simulink library "pwrsys"  (R2018a)
settings: Solver=VariableStepAuto  StartTime=0.0  StopTime=10.0  RelTol=1e-3
values from neighbouring files (symbols this model uses):
  Ts = Ts_c    (= 1e-07)    [PlantStateEquations_abc_Script.m]
undefined symbols (not defined in the file or in its folder): D1, Delta, DiscIntNeverNeededParam, ESS, f_LPF_noise, fn, fsw, grid, gt1, Iap, Kp, PCC, Refmax, Refmin, sim, SIMU, Sn, tctrl, Ti, Ts_control, Ts_PWM, Uabp, Uanp, WT, X, zeta
libraries: $bdroot x71, powerlib x59, powerlib_meascontrol x49, peTransforms x20, PhD_Library x1, sps_avr x1
(part 3 of 4)

== system pwrsys/Transformations/abc_dq ==
  vabc : Inport
  iabc : Inport  Port=2
  wt : Inport  Port=3
  Bus Creator : BusCreator  Inputs=4
  Digital first order LPF : $bdroot/Basic Blocks/Digital first order LPF  Ts=Ts  fcutout=fcutoutv
  Digital first order LPF1 : $bdroot/Basic Blocks/Digital first order LPF  Ts=Ts  fcutout=fcutouti
  Rate Transition1 : RateTransition  OutPortSampleTime=Ts
  Rate Transition2 : RateTransition  OutPortSampleTime=Ts
  Rate Transition4 : RateTransition  OutPortSampleTime=Ts
  Second-Order Filter1 : powerlib_meascontrol/Filters/Second-Order Filter  FilterType=Bandstop (Notch)  Fo=fn  Zeta=zeta  Ts=Ts  Initialize=off  Vac_Init="[0,  0,  60]"  Vdc_Init=0  PlotResponse=off  FreqRange=[0, 1000, 0.1]
      settings: SourceProductName=Simscape Power Systems  SourceProductBaseCode=PS
  Second-Order Filter5 : powerlib_meascontrol/Filters/Second-Order Filter  FilterType=Bandstop (Notch)  Fo=fn  Zeta=zeta  Ts=Ts  Initialize=off  Vac_Init="[0,  0,  60]"  Vdc_Init=0  PlotResponse=off  FreqRange=[0, 1000, 0.1]
      settings: SourceProductName=Simscape Power Systems  SourceProductBaseCode=PS
  Selector4 : Selector  InputPortWidth=3  IndexOptions=Index vector (dialog)  Indices=[1 2]  OutputSizes=1
  Selector5 : Selector  InputPortWidth=3  IndexOptions=Index vector (dialog)  Indices=[1 2]  OutputSizes=1
  abc to dq0 : powerlib_meascontrol/Transformations/abc to dq0  Alignment=90 degrees behind phase A axis
  abc to dq1 : powerlib_meascontrol/Transformations/abc to dq0  Alignment=90 degrees behind phase A axis
  vdq : Outport
  idq : Outport  Port=2
  m : Outport  Port=3
  wires:
  abc to dq1/1 -> Selector4/1
  Selector5/1 -> Digital first order LPF/1, Bus Creator/1  "vdq_unfilt"
  Rate Transition1/1 -> abc to dq0/1
  Rate Transition2/1 -> abc to dq1/2, abc to dq0/2
  Selector4/1 -> Bus Creator/2, Digital first order LPF1/1  "idq_unfilt"
  Rate Transition4/1 -> abc to dq1/1
  abc to dq0/1 -> Selector5/1
  Bus Creator/1 -> m/1
  Second-Order Filter5/1 -> vdq/1, Bus Creator/3  "vdq"
  wt/1 -> Rate Transition2/1
  vabc/1 -> Rate Transition1/1
  iabc/1 -> Rate Transition4/1
  Digital first order LPF1/1 -> Second-Order Filter1/1  "idq"
  Digital first order LPF/1 -> Second-Order Filter5/1  "vdq"
  Second-Order Filter1/1 -> Bus Creator/4, idq/1  "idq"

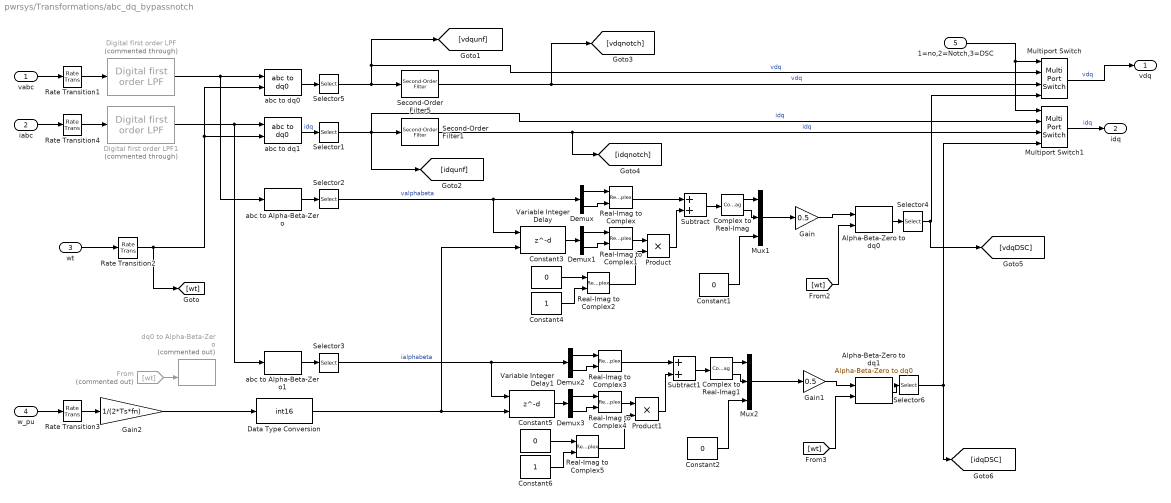
== system pwrsys/Transformations/abc_dq_bypassnotch ==
  vabc : Inport
  iabc : Inport  Port=2
  wt : Inport  Port=3
  w_pu : Inport  Port=4
  1=no,2=Notch,3=DSC : Inport  Port=5
  Alpha-Beta-Zero to dq0 : powerlib_meascontrol/Transformations/Alpha-Beta-Zero to dq0  Alignment=90 degrees behind phase A axis
      settings: SourceProductName=Simscape Power Systems
  Alpha-Beta-Zero to dq1 : powerlib_meascontrol/Transformations/Alpha-Beta-Zero to dq0  Alignment=90 degrees behind phase A axis
      settings: SourceProductName=Simscape Power Systems
  Complex to Real-Imag : ComplexToRealImag
  Complex to Real-Imag1 : ComplexToRealImag
  Constant{1..3,5} (4 alike) : Constant  Value=0
  Constant4 : Constant
  Constant6 : Constant
  Data Type Conversion : DataTypeConversion  OutDataTypeStr=int16  RndMeth=Round  SaturateOnIntegerOverflow=on
  Demux{,1..3} (4 alike) : Demux  Outputs=2
  Digital first order LPF : $bdroot/Basic Blocks/Digital first order LPF  Commented=through  Ts=Ts  fcutout=fcutoutv
  Digital first order LPF1 : $bdroot/Basic Blocks/Digital first order LPF  Commented=through  Ts=Ts  fcutout=fcutouti
  From : From  Commented=on  GotoTag=wt
  Gain : Gain  Gain=0.5
  Gain1 : Gain  Gain=0.5
  Gain2 : Gain  Gain=1/(2*Ts*fn)
  Multiport Switch : MultiPortSwitch
  Multiport Switch1 : MultiPortSwitch
  Mux1 : Mux  Inputs=[1 1 1]
  Mux2 : Mux  Inputs=[1 1 1]
  Product : Product
  Product1 : Product
  Rate Transition1 : RateTransition  OutPortSampleTime=Ts
  Rate Transition2 : RateTransition  OutPortSampleTime=Ts
  Rate Transition3 : RateTransition  InitialCondition=1  OutPortSampleTime=Ts
  Rate Transition4 : RateTransition  OutPortSampleTime=Ts
  Real-Imag to Complex{,1..5} (6 alike) : RealImagToComplex
  Second-Order Filter1 : powerlib_meascontrol/Filters/Second-Order Filter  FilterType=Bandstop (Notch)  Fo=fn  Zeta=zeta  Ts=Ts  Initialize=off  Vac_Init="[0,  0,  60]"  Vdc_Init=0  PlotResponse=off  FreqRange=[0, 1000, 0.1]
      settings: SourceProductName=Simscape Power Systems  SourceProductBaseCode=PS
  Second-Order Filter5 : powerlib_meascontrol/Filters/Second-Order Filter  FilterType=Bandstop (Notch)  Fo=fn  Zeta=zeta  Ts=Ts  Initialize=off  Vac_Init="[0,  0,  60]"  Vdc_Init=0  PlotResponse=off  FreqRange=[0, 1000, 0.1]
      settings: SourceProductName=Simscape Power Systems  SourceProductBaseCode=PS
  Selector{1..6} (6 alike) : Selector  InputPortWidth=3  IndexOptions=Index vector (dialog)  Indices=[1 2]  OutputSizes=1
  Subtract : Sum
  Subtract1 : Sum
  Variable Integer Delay : Delay  DelayLengthSource=Input port  DelayLength=200  DelayLengthUpperLimit=500  SampleTime=Ts
      settings: InputPortMap=u0,p1
  Variable Integer Delay1 : Delay  DelayLengthSource=Input port  DelayLength=200  DelayLengthUpperLimit=500  SampleTime=Ts
      settings: InputPortMap=u0,p1
  abc to Alpha-Beta-Zero : powerlib_meascontrol/Transformations/abc to Alpha-Beta-Zero
      settings: SourceProductName=Simscape Power Systems
  abc to Alpha-Beta-Zero1 : powerlib_meascontrol/Transformations/abc to Alpha-Beta-Zero
      settings: SourceProductName=Simscape Power Systems
  abc to dq0 : powerlib_meascontrol/Transformations/abc to dq0  Alignment=90 degrees behind phase A axis
  abc to dq1 : powerlib_meascontrol/Transformations/abc to dq0  Alignment=90 degrees behind phase A axis
  dq0 to Alpha-Beta-Zero : powerlib_meascontrol/Transformations/dq0 to Alpha-Beta-Zero  Commented=on  Alignment=90 degrees behind phase A axis
      settings: SourceProductName=Simscape Power Systems  SourceProductBaseCode=PS
  vdq : Outport
  idq : Outport  Port=2
  wires:
  Rate Transition1/1 -> Digital first order LPF/1
  Rate Transition2/1 -> [wt], abc to dq1/2, abc to dq0/2
  Rate Transition4/1 -> Digital first order LPF1/1
  wt/1 -> Rate Transition2/1
  abc to dq1/1 -> Selector1/1  "idq"
  Selector5/1 -> Second-Order Filter5/1, [vdqunf], Multiport Switch/2  "vdq"
  Second-Order Filter5/1 -> [vdqnotch], Multiport Switch/3  "vdq"
  Second-Order Filter1/1 -> [idqnotch], Multiport Switch1/3  "idq"
  abc to dq0/1 -> Selector5/1
  Selector1/1 -> [idqunf], Second-Order Filter1/1, Multiport Switch1/2  "idq"
  abc to Alpha-Beta-Zero/1 -> Selector2/1
  abc to Alpha-Beta-Zero1/1 -> Selector3/1
  Gain2/1 -> Data Type Conversion/1
  From/1 -> dq0 to Alpha-Beta-Zero/2
  [wt] -> Alpha-Beta-Zero to dq0/2
  Alpha-Beta-Zero to dq0/1 -> Selector4/1
  Selector4/1 -> [vdqDSC], Multiport Switch/4
  Selector6/1 -> [idqDSC], Multiport Switch1/4
  [wt] -> Alpha-Beta-Zero to dq1/2
  Selector3/1 -> Demux2/1, Variable Integer Delay1/1  "ialphabeta"
  Alpha-Beta-Zero to dq1/1 -> Selector6/1
  Gain/1 -> Alpha-Beta-Zero to dq0/1
  Gain1/1 -> Alpha-Beta-Zero to dq1/1
  Variable Integer Delay/1 -> Demux1/1
  Constant1/1 -> Mux1/3
  Complex to Real-Imag/2 -> Mux1/2
  Constant4/1 -> Real-Imag to Complex2/2
  Complex to Real-Imag/1 -> Mux1/1
  Subtract/1 -> Complex to Real-Imag/1
  Real-Imag to Complex/1 -> Subtract/1
  Demux1/2 -> Real-Imag to Complex1/2
  Real-Imag to Complex1/1 -> Product/1
  Product/1 -> Subtract/2
  Real-Imag to Complex2/1 -> Product/2
  Constant3/1 -> Real-Imag to Complex2/1
  Demux1/1 -> Real-Imag to Complex1/1
  Demux/2 -> Real-Imag to Complex/2
  Demux/1 -> Real-Imag to Complex/1
  Selector2/1 -> Demux/1, Variable Integer Delay/1  "valphabeta"
  Mux1/1 -> Gain/1
  Mux2/1 -> Gain1/1
  Demux2/1 -> Real-Imag to Complex3/1
  Constant5/1 -> Real-Imag to Complex5/1
  Real-Imag to Complex5/1 -> Product1/2
  Demux3/1 -> Real-Imag to Complex4/1
  Product1/1 -> Subtract1/2
  Demux2/2 -> Real-Imag to Complex3/2
  Demux3/2 -> Real-Imag to Complex4/2
  Real-Imag to Complex3/1 -> Subtract1/1
  Constant6/1 -> Real-Imag to Complex5/2
  Real-Imag to Complex4/1 -> Product1/1
  Complex to Real-Imag1/1 -> Mux2/1
  Constant2/1 -> Mux2/3
  Complex to Real-Imag1/2 -> Mux2/2
  Variable Integer Delay1/1 -> Demux3/1
  Subtract1/1 -> Complex to Real-Imag1/1
  Digital first order LPF/1 -> abc to Alpha-Beta-Zero/1, abc to dq0/1
  Digital first order LPF1/1 -> abc to Alpha-Beta-Zero1/1, abc to dq1/1
  w_pu/1 -> Rate Transition3/1
  Rate Transition3/1 -> Gain2/1
  vabc/1 -> Rate Transition1/1
  iabc/1 -> Rate Transition4/1
  Data Type Conversion/1 -> Variable Integer Delay1/2, Variable Integer Delay/2
  Multiport Switch/1 -> vdq/1  "vdq"
  Multiport Switch1/1 -> idq/1  "idq"
  1=no,2=Notch,3=DSC/1 -> Multiport Switch1/1, Multiport Switch/1

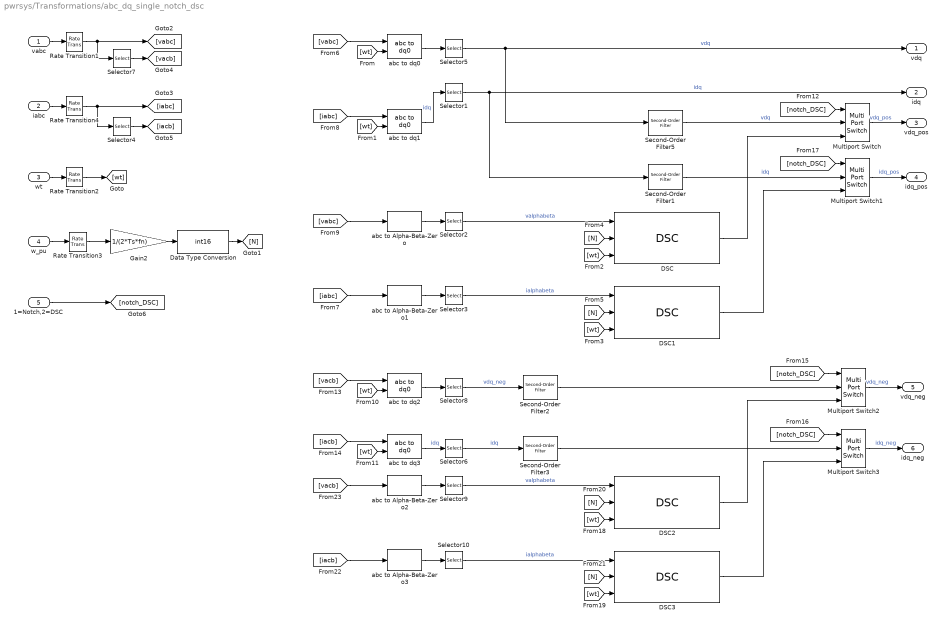
== system pwrsys/Transformations/abc_dq_single_notch_dsc ==
  vabc : Inport
  iabc : Inport  Port=2
  wt : Inport  Port=3
  w_pu : Inport  Port=4
  1=Notch,2=DSC : Inport  Port=5
  DSC{,1..3} (4 alike) : $bdroot/Basic Blocks/DSC
  Data Type Conversion : DataTypeConversion  OutDataTypeStr=int16  RndMeth=Round  SaturateOnIntegerOverflow=on
  Gain2 : Gain  Gain=1/(2*Ts*fn)
  Multiport Switch{,1..3} (4 alike) : MultiPortSwitch  Inputs=2
  Rate Transition1 : RateTransition  OutPortSampleTime=Ts
  Rate Transition2 : RateTransition  OutPortSampleTime=Ts
  Rate Transition3 : RateTransition  InitialCondition=1  OutPortSampleTime=Ts
  Rate Transition4 : RateTransition  OutPortSampleTime=Ts
  Second-Order Filter{1..3,5} (4 alike) : powerlib_meascontrol/Filters/Second-Order Filter  FilterType=Bandstop (Notch)  Fo=fn  Zeta=zeta  Ts=Ts  Initialize=off  Vac_Init="[0,  0,  60]"  Vdc_Init=0  PlotResponse=off  FreqRange=[0, 1000, 0.1]
      settings: SourceProductName=Simscape Power Systems  SourceProductBaseCode=PS
  Selector{1..3,5..6,8..10} (8 alike) : Selector  InputPortWidth=3  IndexOptions=Index vector (dialog)  Indices=[1 2]  OutputSizes=1
  Selector4 : Selector  InputPortWidth=3  IndexOptions=Index vector (dialog)  Indices=[1 3 2]  OutputSizes=1
  Selector7 : Selector  InputPortWidth=3  IndexOptions=Index vector (dialog)  Indices=[1 3 2]  OutputSizes=1
  abc to Alpha-Beta-Zero{,1..3} (4 alike) : powerlib_meascontrol/Transformations/abc to Alpha-Beta-Zero
      settings: SourceProductName=Simscape Power Systems
  abc to dq{0..3} (4 alike) : powerlib_meascontrol/Transformations/abc to dq0  Alignment=90 degrees behind phase A axis
  vdq : Outport
  idq : Outport  Port=2
  vdq_pos : Outport  Port=3
  idq_pos : Outport  Port=4
  vdq_neg : Outport  Port=5
  idq_neg : Outport  Port=6
  wires:
  wt/1 -> Rate Transition2/1
  abc to dq1/1 -> Selector1/1  "idq"
  Selector5/1 -> vdq/1, Second-Order Filter5/1  "vdq"
  abc to dq0/1 -> Selector5/1
  Selector1/1 -> idq/1, Second-Order Filter1/1  "idq"
  abc to Alpha-Beta-Zero/1 -> Selector2/1
  abc to Alpha-Beta-Zero1/1 -> Selector3/1
  Gain2/1 -> Data Type Conversion/1
  DSC/1 -> Multiport Switch/3
  Selector3/1 -> DSC1/1  "ialphabeta"
  [vabc] -> abc to dq0/1
  [iabc] -> abc to dq1/1
  w_pu/1 -> Rate Transition3/1
  Rate Transition3/1 -> Gain2/1
  vabc/1 -> Rate Transition1/1
  iabc/1 -> Rate Transition4/1
  Selector2/1 -> DSC/1  "valphabeta"
  Second-Order Filter5/1 -> Multiport Switch/2  "vdq"
  Second-Order Filter1/1 -> Multiport Switch1/2  "idq"
  DSC1/1 -> Multiport Switch1/3
  Multiport Switch/1 -> vdq_pos/1  "vdq_pos"
  Multiport Switch1/1 -> idq_pos/1  "idq_pos"
  Rate Transition2/1 -> [wt]
  [wt] -> abc to dq0/2
  [wt] -> abc to dq1/2
  [wt] -> DSC/3
  [wt] -> DSC1/3
  [N] -> DSC/2
  [N] -> DSC1/2
  Data Type Conversion/1 -> [N]
  Rate Transition1/1 -> Selector7/1, [vabc]
  Selector7/1 -> [vacb]
  Rate Transition4/1 -> Selector4/1, [iabc]
  Selector4/1 -> [iacb]
  [vabc] -> abc to Alpha-Beta-Zero/1
  [iabc] -> abc to Alpha-Beta-Zero1/1
  [wt] -> abc to dq3/2
  abc to dq2/1 -> Selector8/1
  Selector8/1 -> Second-Order Filter2/1  "vdq_neg"
  [vacb] -> abc to dq2/1
  [wt] -> abc to dq2/2
  abc to dq3/1 -> Selector6/1  "idq"
  [iacb] -> abc to dq3/1
  1=Notch,2=DSC/1 -> [notch_DSC]
  Multiport Switch2/1 -> vdq_neg/1  "vdq_neg"
  Multiport Switch3/1 -> idq_neg/1  "idq_neg"
  Second-Order Filter2/1 -> Multiport Switch2/2
  [notch_DSC] -> Multiport Switch2/1
  [notch_DSC] -> Multiport Switch3/1
  [notch_DSC] -> Multiport Switch/1
  [notch_DSC] -> Multiport Switch1/1
  Selector6/1 -> Second-Order Filter3/1  "idq"
  Second-Order Filter3/1 -> Multiport Switch3/2
  abc to Alpha-Beta-Zero3/1 -> Selector10/1
  Selector10/1 -> DSC3/1  "ialphabeta"
  abc to Alpha-Beta-Zero2/1 -> Selector9/1
  [iacb] -> abc to Alpha-Beta-Zero3/1
  [wt] -> DSC2/3
  [vacb] -> abc to Alpha-Beta-Zero2/1
  DSC2/1 -> Multiport Switch2/3
  Selector9/1 -> DSC2/1  "valphabeta"
  [N] -> DSC3/2
  [N] -> DSC2/2
  DSC3/1 -> Multiport Switch3/3
  [wt] -> DSC3/3

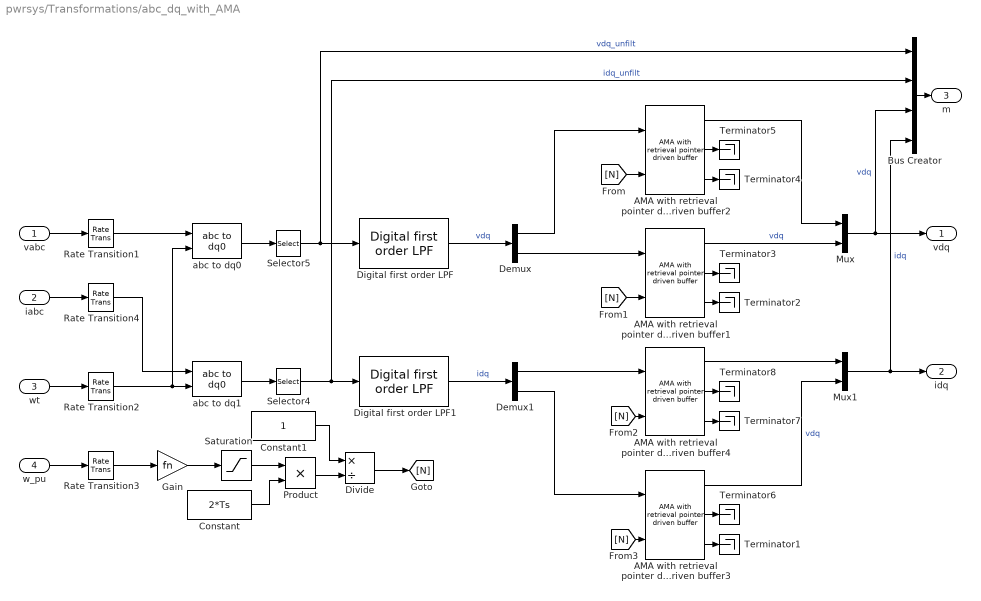
== system pwrsys/Transformations/abc_dq_with_AMA ==
  vabc : Inport
  iabc : Inport  Port=2
  wt : Inport  Port=3
  w_pu : Inport  Port=4
  AMA with retrieval pointer driven buffer{1..4} (4 alike) : $bdroot/Adaptive Moving Averages/AMA with retrieval pointer driven buffer  NbSize=1/(2*fmin*Ts)  Ts=Ts
  Bus Creator : BusCreator  Inputs=4
  Constant : Constant  Value=2*Ts
  Constant1 : Constant
  Demux : Demux  Outputs=2
  Demux1 : Demux  Outputs=2
  Digital first order LPF : $bdroot/Basic Blocks/Digital first order LPF  Ts=Ts  fcutout=fcutoutv
  Digital first order LPF1 : $bdroot/Basic Blocks/Digital first order LPF  Ts=Ts  fcutout=fcutouti
  Divide : Product  Inputs=*/
  Gain : Gain  Gain=fn
  Mux : Mux  Inputs=2
  Mux1 : Mux  Inputs=2
  Product : Product
  Rate Transition1 : RateTransition  OutPortSampleTime=Ts
  Rate Transition2 : RateTransition  OutPortSampleTime=Ts
  Rate Transition3 : RateTransition  InitialCondition=1  OutPortSampleTime=Ts
  Rate Transition4 : RateTransition  OutPortSampleTime=Ts
  Saturation : Saturate  UpperLimit=fmax  LowerLimit=fmin
  Selector4 : Selector  InputPortWidth=3  IndexOptions=Index vector (dialog)  Indices=[1 2]  OutputSizes=1
  Selector5 : Selector  InputPortWidth=3  IndexOptions=Index vector (dialog)  Indices=[1 2]  OutputSizes=1
  Terminator{1..8} (8 alike) : Terminator
  abc to dq0 : powerlib_meascontrol/Transformations/abc to dq0  Alignment=90 degrees behind phase A axis
  abc to dq1 : powerlib_meascontrol/Transformations/abc to dq0  Alignment=90 degrees behind phase A axis
  vdq : Outport
  idq : Outport  Port=2
  m : Outport  Port=3
  wires:
  Digital first order LPF/1 -> Demux/1  "vdq"
  abc to dq1/1 -> Selector4/1
  Mux1/1 -> Bus Creator/4, idq/1  "idq"
  Selector5/1 -> Digital first order LPF/1, Bus Creator/1  "vdq_unfilt"
  Rate Transition1/1 -> abc to dq0/1
  Rate Transition2/1 -> abc to dq0/2, abc to dq1/2
  Selector4/1 -> Bus Creator/2, Digital first order LPF1/1  "idq_unfilt"
  Rate Transition4/1 -> abc to dq1/1
  abc to dq0/1 -> Selector5/1
  Bus Creator/1 -> m/1
  Mux/1 -> Bus Creator/3, vdq/1  "vdq"
  wt/1 -> Rate Transition2/1
  vabc/1 -> Rate Transition1/1
  iabc/1 -> Rate Transition4/1
  AMA with retrieval pointer driven buffer1/3 -> Terminator2/1
  AMA with retrieval pointer driven buffer1/2 -> Terminator3/1
  w_pu/1 -> Rate Transition3/1
  Rate Transition3/1 -> Gain/1
  Gain/1 -> Saturation/1
  Saturation/1 -> Product/1
  Constant/1 -> Product/2
  Product/1 -> Divide/2
  Constant1/1 -> Divide/1
  Divide/1 -> [N]
  Demux/1 -> AMA with retrieval pointer driven buffer2/1
  Demux/2 -> AMA with retrieval pointer driven buffer1/1
  AMA with retrieval pointer driven buffer2/3 -> Terminator4/1
  AMA with retrieval pointer driven buffer2/2 -> Terminator5/1
  AMA with retrieval pointer driven buffer2/1 -> Mux/1
  AMA with retrieval pointer driven buffer1/1 -> Mux/2  "vdq"
  AMA with retrieval pointer driven buffer3/1 -> Mux1/2  "vdq"
  AMA with retrieval pointer driven buffer4/2 -> Terminator8/1
  Demux1/1 -> AMA with retrieval pointer driven buffer4/1
  Demux1/2 -> AMA with retrieval pointer driven buffer3/1
  AMA with retrieval pointer driven buffer4/3 -> Terminator7/1
  AMA with retrieval pointer driven buffer3/3 -> Terminator1/1
  AMA with retrieval pointer driven buffer4/1 -> Mux1/1
  AMA with retrieval pointer driven buffer3/2 -> Terminator6/1
  Digital first order LPF1/1 -> Demux1/1  "idq"
  [N] -> AMA with retrieval pointer driven buffer2/2
  [N] -> AMA with retrieval pointer driven buffer1/2
  [N] -> AMA with retrieval pointer driven buffer4/2
  [N] -> AMA with retrieval pointer driven buffer3/2

== system pwrsys/Transformations/dqz to xyz ==
  note: Inverse Park transform
  dqz : Inport
  scwt : Inport  Port=2
  Demux : Demux  Outputs=3
  Demux1 : Demux  Outputs=2
  Mux : Mux  Inputs=3
  Product{4..7} (4 alike) : Product
  Sum1 : Sum  Inputs=+-
  Sum2 : Sum
  xyz : Outport
  wires:
  dqz/1 -> Demux/1
  Demux/1 -> Product7/2, Product4/2  "d"
  Demux1/2 -> Product4/1, Product6/1
  Product5/1 -> Sum1/2
  Product4/1 -> Sum1/1
  Demux1/1 -> Product7/1, Product5/2
  Demux/2 -> Product6/2, Product5/1  "q"
  scwt/1 -> Demux1/1
  Product6/1 -> Sum2/1
  Product7/1 -> Sum2/2
  Mux/1 -> xyz/1
  Demux/3 -> Mux/3  "z"
  Sum2/1 -> Mux/2  "y"
  Sum1/1 -> Mux/1  "x"

== system pwrsys/Transformations/xyz to abc ==
  note: Inverse Clark Transform
  xyz : Inport
  Demux : Demux  Outputs=3
  Gain : Gain  Gain=d
  Gain1 : Gain  Gain=c
  Gain2 : Gain  Gain=b
  Gain3 : Gain  Gain=a
  Mux : Mux  Inputs=3
  Sum3 : Sum  Inputs=-+
  Sum4 : Sum  Inputs=-+
  Sum5 : Sum
  Sum6 : Sum
  abc : Outport
  wires:
  xyz/1 -> Demux/1
  Demux/2 -> Gain2/1  "y"
  Demux/1 -> Gain3/1, Gain1/1  "x"
  Demux/3 -> Gain/1  "z"
  Gain1/1 -> Sum3/1
  Gain/1 -> Sum6/2, Sum3/2  "A"
  Gain2/1 -> Sum5/1, Sum4/1
  Sum3/1 -> Sum5/2, Sum4/2  "B"
  Sum4/1 -> Mux/3  "c"
  Sum5/1 -> Mux/2  "b"
  Sum6/1 -> Mux/1  "a"
  Gain3/1 -> Sum6/1
  Mux/1 -> abc/1

== system pwrsys/Transformations/xyz to dqz ==
  note: Park transform
  xyz : Inport
  scwt : Inport  Port=2
  Demux : Demux  Outputs=3
  Demux1 : Demux  Outputs=2
  Mux : Mux  Inputs=3
  Product{4..7} (4 alike) : Product
  Sum1 : Sum
  Sum2 : Sum  Inputs=+-
  dqz : Outport
  wires:
  Sum1/1 -> Mux/1  "d"
  Sum2/1 -> Mux/2  "q"
  Demux/3 -> Mux/3  "z"
  Mux/1 -> dqz/1
  Product7/1 -> Sum2/2
  Product6/1 -> Sum2/1
  scwt/1 -> Demux1/1
  Demux/2 -> Product5/1, Product6/2  "y"
  Demux1/1 -> Product5/2, Product7/1
  Product4/1 -> Sum1/1
  Product5/1 -> Sum1/2
  Demux1/2 -> Product6/1, Product4/1
  Demux/1 -> Product4/2, Product7/2  "x"
  xyz/1 -> Demux/1

== system pwrsys/Voltage Sources/Balanced_3_phase_Vsource ==
  amp_pu : Inport
  time_s : Inport  Port=2
  phase_deg : Inport  Port=3
  pos1_neg-1 : Inport  Port=4
  f_pu : Inport  Port=5
  Add3 : Sum  Inputs=+-+
  Add4 : Sum  Inputs=+++
  Add5 : Sum
  Amplitude_Base : Constant  Value=BaseAmp
  Bus Creator : BusCreator  Inputs=3
  Constant : Constant  Value=2*pi
  Constant4 : Constant  Value=2*pi/3
  Constant6 : Constant  Value=2*pi
  Controlled Voltage Source : powerlib/Electrical Sources/Controlled Voltage Source  Initialize=off  Source_Type=AC  Amplitude=ESS.LSC.Ub*(2/3)^0.5  Phase=0  Frequency=PCC.fn  Measurements=None
  Controlled Voltage Source1 : powerlib/Electrical Sources/Controlled Voltage Source  Initialize=off  Source_Type=AC  Amplitude=ESS.LSC.Ub*(2/3)^0.5  Phase=-120  Frequency=PCC.fn  Measurements=None
  Controlled Voltage Source2 : powerlib/Electrical Sources/Controlled Voltage Source  Initialize=off  Source_Type=AC  Amplitude=ESS.LSC.Ub*(2/3)^0.5  Phase=120  Frequency=PCC.fn  Measurements=None
  Gain : Gain  Gain=pi/180
  Gain1 : Gain  Gain=fn
  Product{1,3..5,8} (5 alike) : Product
  Product2 : Product  Inputs=3
  Relay : Relay  OnSwitchValue=0  OffSwitchValue=-0.1  OffOutputValue=-1
  Trigonometric Function3 : Trigonometry
  Trigonometric Function4 : Trigonometry
  Trigonometric Function5 : Trigonometry
  mod : Math  Operator=mod  SaturateOnIntegerOverflow=on
  Va+ : PMIOPort  Side=Right
  Vb+ : PMIOPort  Port=2  Side=Right
  Vc+ : PMIOPort  Port=3  Side=Right
  Va- : PMIOPort  Port=4  Side=Right
  Vb- : PMIOPort  Port=5  Side=Right
  Vc- : PMIOPort  Port=6  Side=Right
  Amp_V : Outport
  phase_rad : Outport  Port=2
  wt_phase_a : Outport  Port=3
  Vabc : Outport  Port=4
  wires:
  Add4/1 -> Trigonometric Function5/1
  Gain/1 -> phase_rad/1, Add4/3, Add3/3, Add5/2  "phase"
  Add3/1 -> Trigonometric Function4/1
  pos1_neg-1/1 -> Relay/1
  Product3/1 -> Bus Creator/1, Controlled Voltage Source/1  "Va"
  amp_pu/1 -> Product1/1
  Product8/1 -> Add3/2, Add4/2
  Product5/1 -> Bus Creator/3, Controlled Voltage Source2/1  "Vc"
  Product4/1 -> Bus Creator/2, Controlled Voltage Source1/1  "Vb"
  Amplitude_Base/1 -> Product1/2
  Constant4/1 -> Product8/1
  Product1/1 -> Product5/1, Product4/1, Product3/1, Amp_V/1  "amp"
  Relay/1 -> Product8/2
  Trigonometric Function3/1 -> Product3/2
  Product2/1 -> Add5/1, Add4/1, Add3/1  "wt"
  Trigonometric Function5/1 -> Product5/2
  Add5/1 -> mod/1, Trigonometric Function3/1
  Trigonometric Function4/1 -> Product4/2
  phase_deg/1 -> Gain/1
  time_s/1 -> Product2/2
  Constant/1 -> Product2/1
  f_pu/1 -> Gain1/1
  Gain1/1 -> Product2/3
  Bus Creator/1 -> Vabc/1
  Constant6/1 -> mod/2
  mod/1 -> wt_phase_a/1
  connections:
  Vb+/RConn1 -- Controlled Voltage Source1/RConn1
  Vc+/RConn1 -- Controlled Voltage Source2/RConn1
  Va+/RConn1 -- Controlled Voltage Source/RConn1
  Va-/RConn1 -- Controlled Voltage Source/LConn1
  Vb-/RConn1 -- Controlled Voltage Source1/LConn1
  Vc-/RConn1 -- Controlled Voltage Source2/LConn1

== system pwrsys/Voltage Sources/DCL_LSC_LCL_Trafo_NoSwitching ==
  Open_Close_Breaker : Inport
  Vabcref : Inport  Port=2
  Bus Creator : BusCreator  Inputs=8
  Cdclink : powerlib/Elements/Parallel RLC Branch  LConnTagsString=a  RConnTagsString=__new0  BranchType=RC  Resistance=1e6  Inductance=0  SetiL0=off  InitialCurrent=0  Capacitance=Cdc  Setx0=on  InitialVoltage=Udc0  Measurements=None
  Controlled Current Source2 : powerlib/Electrical Sources/Controlled Current Source  Initialize=on  Source_Type=DC  Amplitude=0  Phase=0  Frequency=50  Measurements=None
  Controlled Voltage Source : powerlib/Electrical Sources/Controlled Voltage Source  Initialize=on  Source_Type=AC  Amplitude=Uab*(2/3)^0.5  Phase=30  Frequency=fn  Measurements=None
  Controlled Voltage Source1 : powerlib/Electrical Sources/Controlled Voltage Source  Initialize=on  Source_Type=AC  Amplitude=Uab*(2/3)^0.5  Phase=30-120  Frequency=fn  Measurements=None
  Controlled Voltage Source2 : powerlib/Electrical Sources/Controlled Voltage Source  Initialize=on  Source_Type=AC  Amplitude=Uab*(2/3)^0.5  Phase=30+120  Frequency=fn  Measurements=None
  Current Measurement : powerlib/Measurements/Current Measurement  PhasorSimulation=off  OutputType=Complex  PSBequivalent=0
  Demux2 : Demux  Outputs=3
  Divide : Product  Inputs=**/
  Dot Product : DotProduct  InputSameDT=on  OutDataTypeStr=Inherit: Inherit via internal rule
  HV : powerlib/Measurements/Three-Phase V-I Measurement  VoltageMeasurement=phase-to-ground  SetLabelV=off  LabelV=vgrid  Vpu=off  VpuLL=off  CurrentMeasurement=yes  SetLabelI=off  LabelI=igrid  Ipu=off  Pbase=sn  Vbase=uab  OutputType=Complex  PhasorSimulation=off  PSBequivalent=0
  High Res Grounding : powerlib/Elements/Three-Phase Parallel RLC Load  LConnTagsString=A|B|C  Configuration=Y (grounded)  NominalVoltage=Uab  Vabc=[1e3 1e3 1e3]  Vabcp=[1e3 1e3 1e3]  NominalFrequency=fn  UnbalancedPower=off  ActivePower=0.001  InductivePower=0  CapacitivePower=0  Pabc=[10e3 9e3 11e3]  QLabc=[100 90 110]  QCabc=[100 90 110]  Pabcp=[10e3 9e3 11e3]  QLabcp=[100 90 110]  QCabcp=[100 90 110]  Measurements=None  LoadType=constant Z
  INV : powerlib/Measurements/Three-Phase V-I Measurement  VoltageMeasurement=phase-to-ground  SetLabelV=off  LabelV=vconv  Vpu=off  VpuLL=off  CurrentMeasurement=yes  SetLabelI=off  LabelI=iconv  Ipu=off  Pbase=sn  Vbase=uab  OutputType=Complex  PhasorSimulation=off  PSBequivalent=0
  LV : powerlib/Measurements/Three-Phase V-I Measurement  VoltageMeasurement=phase-to-ground  SetLabelV=off  LabelV=vgrid  Vpu=off  VpuLL=off  CurrentMeasurement=yes  SetLabelI=off  LabelI=igrid  Ipu=off  Pbase=sn  Vbase=uab  OutputType=Complex  PhasorSimulation=off  PSBequivalent=0
  La_DVR1 : powerlib/Elements/Series RLC Branch  LConnTagsString=__new0  RConnTagsString=__new0  BranchType=RL  Resistance=Rf1  Inductance=Lf1  SetiL0=off  InitialCurrent=0  Capacitance=1.0  Setx0=off  InitialVoltage=0  Measurements=None
  La_DVR2 : powerlib/Elements/Series RLC Branch  LConnTagsString=__new0  RConnTagsString=__new0  BranchType=RL  Resistance=Rf1  Inductance=Lf1  SetiL0=off  InitialCurrent=0  Capacitance=1.0  Setx0=off  InitialVoltage=0  Measurements=None
  La_DVR3 : powerlib/Elements/Series RLC Branch  LConnTagsString=__new0  RConnTagsString=__new0  BranchType=RL  Resistance=Rf1  Inductance=Lf1  SetiL0=off  InitialCurrent=0  Capacitance=1.0  Setx0=off  InitialVoltage=0  Measurements=None
  La_DVR4 : powerlib/Elements/Series RLC Branch  LConnTagsString=__new0  RConnTagsString=__new0  BranchType=RC  Resistance=Rc  Inductance=Lf1  SetiL0=off  InitialCurrent=0  Capacitance=Cf  Setx0=off  InitialVoltage=0  Measurements=None
  La_DVR5 : powerlib/Elements/Series RLC Branch  LConnTagsString=__new0  RConnTagsString=__new0  BranchType=RC  Resistance=Rc  Inductance=Lf1  SetiL0=off  InitialCurrent=0  Capacitance=Cf  Setx0=off  InitialVoltage=0  Measurements=None
  La_DVR6 : powerlib/Elements/Series RLC Branch  LConnTagsString=__new0  RConnTagsString=__new0  BranchType=RC  Resistance=Rc  Inductance=Lf1  SetiL0=off  InitialCurrent=0  Capacitance=Cf  Setx0=off  InitialVoltage=0  Measurements=None
  Saturation : Saturate  UpperLimit=10*Uab*sqrt(2/3)  LowerLimit=0.01*Uab*sqrt(2/3)
  Step6 : Step  Time=Tstart  SampleTime=0
  Three-Phase Transformer (Two Windings) : powerlib/Elements/Three-Phase Transformer (Two Windings)  Winding1Connection=Y  Winding2Connection=Delta (D1)  CoreType=Three-limb core (core-type)  SetSaturation=off  Hysteresis=off  DataFile='hysteresis'  SetInitialFlux=off  Measurements=None  UNITS=pu  NominalPower=[ Sn , fn ]  Winding1=[ Uhv_ab , rf2/2 , lf2/2 ]  Winding2=[ Uab , rf2/2 , lf2/2 ]  Rm=500  Lm=500  L0=0.5  Saturation=[ 0,0 ; 0.0024,1.2 ; 1.0,1.52 ]  InitialFluxes=[0 0 0]  MoreParameters=off  BreakLoop=off  DataType=off  TransfoNumber=1
  Three-Phase Breaker : powerlib/Elements/Three-Phase Breaker  InitialState=open  SwitchA=on  SwitchB=on  SwitchC=on  SwitchTimes="[1/60  5/60]"  External=on  BreakerResistance=0.01  SnubberResistance=1e6  SnubberCapacitance=inf  Measurements=None
  Unit Delay1 : UnitDelay  SampleTime=Tsm
  Voltage Measurement : powerlib/Measurements/Voltage Measurement  PhasorSimulation=off  OutputType=Magnitude  PSBequivalent=0
  A : PMIOPort  Side=Right
  B : PMIOPort  Port=2  Side=Right
  C : PMIOPort  Port=3  Side=Right
  P : PMIOPort  Port=4  Side=Left
  N : PMIOPort  Port=5  Side=Left
  m : Outport
  wires:
  HV/2 -> Bus Creator/4  "HV_Iabc"
  LV/1 -> [LV_Vabc], Bus Creator/5  "LV_Vabc"
  INV/1 -> [INV_Vabc], Bus Creator/7  "INV_Vabc"
  INV/2 -> [INV_Iabc], Bus Creator/8  "INV_Iabc"
  HV/1 -> Bus Creator/3  "HV_Vabc"
  LV/2 -> Bus Creator/6  "LV_Iabc"
  Bus Creator/1 -> m/1
  Open_Close_Breaker/1 -> Three-Phase Breaker/1
  Vabcref/1 -> Demux2/1
  Demux2/1 -> Controlled Voltage Source/1  "Va"
  Demux2/2 -> Controlled Voltage Source1/1  "Vb"
  Demux2/3 -> Controlled Voltage Source2/1  "Vc"
  Voltage Measurement/1 -> [Vdc], Saturation/1  "Vdc"
  Saturation/1 -> Divide/3
  Dot Product/1 -> Divide/2
  Divide/1 -> Unit Delay1/1
  [INV_Vabc] -> Dot Product/1
  [INV_Iabc] -> Dot Product/2
  [Vdc] -> Bus Creator/1  "INV_Vdc"
  [Idc] -> Bus Creator/2  "INV_Idc"
  Unit Delay1/1 -> Controlled Current Source2/1
  Step6/1 -> Divide/1
  Current Measurement/1 -> [Idc]
  connections:
  La_DVR1/LConn1 -- INV/RConn1
  LV/RConn1 -- Three-Phase Transformer (Two Windings)/RConn1 -- High Res Grounding/LConn1
  La_DVR1/RConn1 -- La_DVR4/RConn1 -- LV/LConn1
  Three-Phase Transformer (Two Windings)/LConn3 -- HV/LConn3
  Three-Phase Transformer (Two Windings)/RConn3 -- LV/RConn3 -- High Res Grounding/LConn3
  La_DVR2/RConn1 -- La_DVR5/RConn1 -- LV/LConn2
  Three-Phase Transformer (Two Windings)/LConn2 -- HV/LConn2
  Three-Phase Transformer (Two Windings)/RConn2 -- LV/RConn2 -- High Res Grounding/LConn2
  Three-Phase Transformer (Two Windings)/LConn1 -- HV/LConn1
  LV/LConn3 -- La_DVR3/RConn1 -- La_DVR6/RConn1
  La_DVR3/LConn1 -- INV/RConn3
  La_DVR5/LConn1 -- La_DVR6/LConn1 -- La_DVR4/LConn1
  La_DVR2/LConn1 -- INV/RConn2
  Three-Phase Breaker/LConn2 -- B/RConn1
  Three-Phase Breaker/RConn2 -- HV/RConn2
  HV/RConn3 -- Three-Phase Breaker/RConn3
  Three-Phase Breaker/LConn3 -- C/RConn1
  HV/RConn1 -- Three-Phase Breaker/RConn1
  Three-Phase Breaker/LConn1 -- A/RConn1
  Controlled Voltage Source2/LConn1 -- Controlled Voltage Source/LConn1 -- Controlled Voltage Source1/LConn1
  INV/LConn1 -- Controlled Voltage Source/RConn1
  Controlled Voltage Source1/RConn1 -- INV/LConn2
  Controlled Voltage Source2/RConn1 -- INV/LConn3
  Voltage Measurement/LConn2 -- Controlled Current Source2/RConn1 -- Cdclink/RConn1 -- N/RConn1
  Controlled Current Source2/LConn1 -- Current Measurement/RConn1 -- Cdclink/LConn1 -- Voltage Measurement/LConn1
  P/RConn1 -- Current Measurement/LConn1

== system pwrsys/Voltage Sources/LSC_LCL_Trafo ==
  Gates : Inport
  Block_IGBTs : Inport  Port=2
  Open_Close_Breaker : Inport  Port=3
  Bus Creator : BusCreator  Inputs=8
  HV : powerlib/Measurements/Three-Phase V-I Measurement  VoltageMeasurement=phase-to-ground  SetLabelV=off  LabelV=vgrid  Vpu=off  VpuLL=off  CurrentMeasurement=yes  SetLabelI=off  LabelI=igrid  Ipu=off  Pbase=sn  Vbase=uab  OutputType=Complex  PhasorSimulation=off  PSBequivalent=0
  High Res Grounding : powerlib/Elements/Three-Phase Parallel RLC Load  LConnTagsString=A|B|C  Configuration=Y (grounded)  NominalVoltage=Uab  Vabc=[1e3 1e3 1e3]  Vabcp=[1e3 1e3 1e3]  NominalFrequency=fn  UnbalancedPower=off  ActivePower=0.001  InductivePower=0  CapacitivePower=0  Pabc=[10e3 9e3 11e3]  QLabc=[100 90 110]  QCabc=[100 90 110]  Pabcp=[10e3 9e3 11e3]  QLabcp=[100 90 110]  QCabcp=[100 90 110]  Measurements=None  LoadType=constant Z
  INV : powerlib/Measurements/Three-Phase V-I Measurement  VoltageMeasurement=phase-to-ground  SetLabelV=off  LabelV=vconv  Vpu=off  VpuLL=off  CurrentMeasurement=yes  SetLabelI=off  LabelI=iconv  Ipu=off  Pbase=sn  Vbase=uab  OutputType=Complex  PhasorSimulation=off  PSBequivalent=0
  INV_DClink : Subsystem
  LSC : powerlib/Power Electronics/Two-Level Converter  ModelType=Switching devices  Ron=1e-3  Rs=1e6  Cs=inf  Vforward=[ 0, 0 ]  Ron_Diode=1e-3  Rs_Diode=1e6  Cs_Diode=inf  Vf_Diode=1e-3  Rs_CurrentSource=inf
      settings: AttributesFormatString=%<ModelType>  SourceProductName=Simscape Power Systems  SourceProductBaseCode=PS
  LV : powerlib/Measurements/Three-Phase V-I Measurement  VoltageMeasurement=phase-to-ground  SetLabelV=off  LabelV=vgrid  Vpu=off  VpuLL=off  CurrentMeasurement=yes  SetLabelI=off  LabelI=igrid  Ipu=off  Pbase=sn  Vbase=uab  OutputType=Complex  PhasorSimulation=off  PSBequivalent=0
  La_DVR1 : powerlib/Elements/Series RLC Branch  LConnTagsString=__new0  RConnTagsString=__new0  BranchType=RL  Resistance=Rf1  Inductance=Lf1  SetiL0=off  InitialCurrent=0  Capacitance=1.0  Setx0=off  InitialVoltage=0  Measurements=None
  La_DVR2 : powerlib/Elements/Series RLC Branch  LConnTagsString=__new0  RConnTagsString=__new0  BranchType=RL  Resistance=Rf1  Inductance=Lf1  SetiL0=off  InitialCurrent=0  Capacitance=1.0  Setx0=off  InitialVoltage=0  Measurements=None
  La_DVR3 : powerlib/Elements/Series RLC Branch  LConnTagsString=__new0  RConnTagsString=__new0  BranchType=RL  Resistance=Rf1  Inductance=Lf1  SetiL0=off  InitialCurrent=0  Capacitance=1.0  Setx0=off  InitialVoltage=0  Measurements=None
  La_DVR4 : powerlib/Elements/Series RLC Branch  LConnTagsString=__new0  RConnTagsString=__new0  BranchType=RC  Resistance=Rc  Inductance=Lf1  SetiL0=off  InitialCurrent=0  Capacitance=Cf  Setx0=off  InitialVoltage=0  Measurements=None
  La_DVR5 : powerlib/Elements/Series RLC Branch  LConnTagsString=__new0  RConnTagsString=__new0  BranchType=RC  Resistance=Rc  Inductance=Lf1  SetiL0=off  InitialCurrent=0  Capacitance=Cf  Setx0=off  InitialVoltage=0  Measurements=None
  La_DVR6 : powerlib/Elements/Series RLC Branch  LConnTagsString=__new0  RConnTagsString=__new0  BranchType=RC  Resistance=Rc  Inductance=Lf1  SetiL0=off  InitialCurrent=0  Capacitance=Cf  Setx0=off  InitialVoltage=0  Measurements=None
  Three-Phase Transformer (Two Windings) : powerlib/Elements/Three-Phase Transformer (Two Windings)  Winding1Connection=Y  Winding2Connection=Delta (D1)  CoreType=Three-limb core (core-type)  SetSaturation=off  Hysteresis=off  DataFile='hysteresis'  SetInitialFlux=off  Measurements=None  UNITS=pu  NominalPower=[ Sn , fn ]  Winding1=[ Uhv_ab , rf2/2 , lf2/2 ]  Winding2=[ Uab , rf2/2 , lf2/2 ]  Rm=500  Lm=500  L0=0.5  Saturation=[ 0,0 ; 0.0024,1.2 ; 1.0,1.52 ]  InitialFluxes=[0 0 0]  MoreParameters=off  BreakLoop=off  DataType=off  TransfoNumber=1
  Three-Phase Breaker : powerlib/Elements/Three-Phase Breaker  InitialState=open  SwitchA=on  SwitchB=on  SwitchC=on  SwitchTimes="[1/60  5/60]"  External=on  BreakerResistance=0.01  SnubberResistance=1e6  SnubberCapacitance=inf  Measurements=None
  "\tP" : PMIOPort  Side=Left
  M : PMIOPort  Port=2  Side=Left
  A : PMIOPort  Port=3  Side=Right
  B : PMIOPort  Port=4  Side=Right
  C : PMIOPort  Port=5  Side=Right
  m : Outport
  wires:
  HV/2 -> Bus Creator/2  "HV_Iabc"
  LV/1 -> Bus Creator/3  "LV_Vabc"
  INV/1 -> Bus Creator/5  "INV_Vabc"
  INV_DClink/2(Idc) -> Bus Creator/8  "Idc"
  INV/2 -> Bus Creator/6  "INV_Iabc"
  Block_IGBTs/1 -> LSC/2
  INV_DClink/1(Vdc) -> Bus Creator/7  "Vdc"
  HV/1 -> Bus Creator/1  "HV_Vabc"
  LV/2 -> Bus Creator/4  "LV_Iabc"
  Bus Creator/1 -> m/1
  Gates/1 -> LSC/1
  Open_Close_Breaker/1 -> Three-Phase Breaker/1
  connections:
  La_DVR1/LConn1 -- INV/RConn1
  LV/RConn1 -- Three-Phase Transformer (Two Windings)/RConn1 -- High Res Grounding/LConn1
  La_DVR1/RConn1 -- La_DVR4/RConn1 -- LV/LConn1
  LSC/LConn3 -- INV/LConn3
  Three-Phase Transformer (Two Windings)/LConn3 -- HV/LConn3
  LSC/LConn2 -- INV/LConn2
  Three-Phase Transformer (Two Windings)/RConn3 -- LV/RConn3 -- High Res Grounding/LConn3
  La_DVR2/RConn1 -- La_DVR5/RConn1 -- LV/LConn2
  Three-Phase Transformer (Two Windings)/LConn2 -- HV/LConn2
  LSC/RConn2 -- INV_DClink/RConn2
  LSC/LConn1 -- INV/LConn1
  LSC/RConn1 -- INV_DClink/RConn1
  Three-Phase Transformer (Two Windings)/RConn2 -- LV/RConn2 -- High Res Grounding/LConn2
  "\tP"/RConn1 -- INV_DClink/LConn1
  Three-Phase Transformer (Two Windings)/LConn1 -- HV/LConn1
  LV/LConn3 -- La_DVR3/RConn1 -- La_DVR6/RConn1
  La_DVR3/LConn1 -- INV/RConn3
  La_DVR5/LConn1 -- La_DVR6/LConn1 -- La_DVR4/LConn1
  La_DVR2/LConn1 -- INV/RConn2
  INV_DClink/LConn2 -- M/RConn1
  Three-Phase Breaker/LConn2 -- B/RConn1
  Three-Phase Breaker/RConn2 -- HV/RConn2
  HV/RConn3 -- Three-Phase Breaker/RConn3
  Three-Phase Breaker/LConn3 -- C/RConn1
  HV/RConn1 -- Three-Phase Breaker/RConn1
  Three-Phase Breaker/LConn1 -- A/RConn1

== system pwrsys/Voltage Sources/LSC_LCL_Trafo_AvgxSwitch ==
  Gates : Inport
  0=Avg_1=Switch : Inport  Port=2
  Open_Close_Breaker : Inport  Port=3
  Vabcref : Inport  Port=4
  Bus Creator : BusCreator  Inputs=8
  Constant : Constant  Value=0
  Constant1 : Constant  Value=0
  Constant2 : Constant
  Constant3 : Constant
  Constant4 : Constant  Value=0
  Controlled Voltage Source : powerlib/Electrical Sources/Controlled Voltage Source  Initialize=off  Source_Type=AC  Amplitude=ESS.LSC.Ub*(2/3)^0.5  Phase=0  Frequency=PCC.fn  Measurements=None
  Controlled Voltage Source1 : powerlib/Electrical Sources/Controlled Voltage Source  Initialize=off  Source_Type=AC  Amplitude=ESS.LSC.Ub*(2/3)^0.5  Phase=-120  Frequency=PCC.fn  Measurements=None
  Controlled Voltage Source2 : powerlib/Electrical Sources/Controlled Voltage Source  Initialize=off  Source_Type=AC  Amplitude=ESS.LSC.Ub*(2/3)^0.5  Phase=120  Frequency=PCC.fn  Measurements=None
  Demux2 : Demux  Outputs=3
  HV : powerlib/Measurements/Three-Phase V-I Measurement  VoltageMeasurement=phase-to-ground  SetLabelV=off  LabelV=vgrid  Vpu=off  VpuLL=off  CurrentMeasurement=yes  SetLabelI=off  LabelI=igrid  Ipu=off  Pbase=sn  Vbase=uab  OutputType=Complex  PhasorSimulation=off  PSBequivalent=0
  High Res Grounding : powerlib/Elements/Three-Phase Parallel RLC Load  LConnTagsString=A|B|C  Configuration=Y (grounded)  NominalVoltage=Uab  Vabc=[1e3 1e3 1e3]  Vabcp=[1e3 1e3 1e3]  NominalFrequency=fn  UnbalancedPower=off  ActivePower=0.001  InductivePower=0  CapacitivePower=0  Pabc=[10e3 9e3 11e3]  QLabc=[100 90 110]  QCabc=[100 90 110]  Pabcp=[10e3 9e3 11e3]  QLabcp=[100 90 110]  QCabcp=[100 90 110]  Measurements=None  LoadType=constant Z
  INV : powerlib/Measurements/Three-Phase V-I Measurement  VoltageMeasurement=phase-to-ground  SetLabelV=off  LabelV=vconv  Vpu=off  VpuLL=off  CurrentMeasurement=yes  SetLabelI=off  LabelI=iconv  Ipu=off  Pbase=sn  Vbase=uab  OutputType=Complex  PhasorSimulation=off  PSBequivalent=0
  INV_DClink : Subsystem
  LSC : powerlib/Power Electronics/Two-Level Converter  ModelType=Switching devices  Ron=1e-3  Rs=1e6  Cs=inf  Vforward=[ 0, 0 ]  Ron_Diode=1e-3  Rs_Diode=1e6  Cs_Diode=inf  Vf_Diode=1e-3  Rs_CurrentSource=inf
      settings: AttributesFormatString=%<ModelType>  SourceProductName=Simscape Power Systems  SourceProductBaseCode=PS
  LV : powerlib/Measurements/Three-Phase V-I Measurement  VoltageMeasurement=phase-to-ground  SetLabelV=off  LabelV=vgrid  Vpu=off  VpuLL=off  CurrentMeasurement=yes  SetLabelI=off  LabelI=igrid  Ipu=off  Pbase=sn  Vbase=uab  OutputType=Complex  PhasorSimulation=off  PSBequivalent=0
  La_DVR1 : powerlib/Elements/Series RLC Branch  LConnTagsString=__new0  RConnTagsString=__new0  BranchType=RL  Resistance=Rf1  Inductance=Lf1  SetiL0=off  InitialCurrent=0  Capacitance=1.0  Setx0=off  InitialVoltage=0  Measurements=None
  La_DVR2 : powerlib/Elements/Series RLC Branch  LConnTagsString=__new0  RConnTagsString=__new0  BranchType=RL  Resistance=Rf1  Inductance=Lf1  SetiL0=off  InitialCurrent=0  Capacitance=1.0  Setx0=off  InitialVoltage=0  Measurements=None
  La_DVR3 : powerlib/Elements/Series RLC Branch  LConnTagsString=__new0  RConnTagsString=__new0  BranchType=RL  Resistance=Rf1  Inductance=Lf1  SetiL0=off  InitialCurrent=0  Capacitance=1.0  Setx0=off  InitialVoltage=0  Measurements=None
  La_DVR4 : powerlib/Elements/Series RLC Branch  LConnTagsString=__new0  RConnTagsString=__new0  BranchType=RC  Resistance=Rc  Inductance=Lf1  SetiL0=off  InitialCurrent=0  Capacitance=Cf  Setx0=off  InitialVoltage=0  Measurements=None
  La_DVR5 : powerlib/Elements/Series RLC Branch  LConnTagsString=__new0  RConnTagsString=__new0  BranchType=RC  Resistance=Rc  Inductance=Lf1  SetiL0=off  InitialCurrent=0  Capacitance=Cf  Setx0=off  InitialVoltage=0  Measurements=None
  La_DVR6 : powerlib/Elements/Series RLC Branch  LConnTagsString=__new0  RConnTagsString=__new0  BranchType=RC  Resistance=Rc  Inductance=Lf1  SetiL0=off  InitialCurrent=0  Capacitance=Cf  Setx0=off  InitialVoltage=0  Measurements=None
  Switch : Switch  Criteria=u2 > Threshold  Threshold=0.5
  Switch1 : Switch  Criteria=u2 > Threshold  Threshold=0.5
  Three-Phase Transformer (Two Windings) : powerlib/Elements/Three-Phase Transformer (Two Windings)  Winding1Connection=Y  Winding2Connection=Delta (D1)  CoreType=Three-limb core (core-type)  SetSaturation=off  Hysteresis=off  DataFile='hysteresis'  SetInitialFlux=off  Measurements=None  UNITS=pu  NominalPower=[ Sn , fn ]  Winding1=[ Uhv_ab , rf2/2 , lf2/2 ]  Winding2=[ Uab , rf2/2 , lf2/2 ]  Rm=500  Lm=500  L0=0.5  Saturation=[ 0,0 ; 0.0024,1.2 ; 1.0,1.52 ]  InitialFluxes=[0 0 0]  MoreParameters=off  BreakLoop=off  DataType=off  TransfoNumber=1
  Three-Phase Breaker : powerlib/Elements/Three-Phase Breaker  InitialState=open  SwitchA=on  SwitchB=on  SwitchC=on  SwitchTimes="[1/60  5/60]"  External=on  BreakerResistance=0.01  SnubberResistance=1e6  SnubberCapacitance=inf  Measurements=None
  Three-Phase Breaker1 : powerlib/Elements/Three-Phase Breaker  InitialState=open  SwitchA=on  SwitchB=on  SwitchC=on  SwitchTimes="[1/60  5/60]"  External=on  BreakerResistance=0.000000000001  SnubberResistance=1e10  SnubberCapacitance=inf  Measurements=None
  Three-Phase Breaker2 : powerlib/Elements/Three-Phase Breaker  InitialState=open  SwitchA=on  SwitchB=on  SwitchC=on  SwitchTimes="[1/60  5/60]"  External=on  BreakerResistance=0.000000000001  SnubberResistance=1e10  SnubberCapacitance=inf  Measurements=None
  "\tP" : PMIOPort  Side=Left
  M : PMIOPort  Port=2  Side=Left
  A : PMIOPort  Port=3  Side=Right
  B : PMIOPort  Port=4  Side=Right
  C : PMIOPort  Port=5  Side=Right
  m : Outport
  wires:
  HV/2 -> Bus Creator/2  "HV_Iabc"
  LV/1 -> Bus Creator/3  "LV_Vabc"
  INV/1 -> Bus Creator/5  "INV_Vabc"
  INV_DClink/2(Idc) -> Bus Creator/8  "Idc"
  INV/2 -> Bus Creator/6  "INV_Iabc"
  INV_DClink/1(Vdc) -> Bus Creator/7  "Vdc"
  HV/1 -> Bus Creator/1  "HV_Vabc"
  LV/2 -> Bus Creator/4  "LV_Iabc"
  Bus Creator/1 -> m/1
  Gates/1 -> LSC/1
  Open_Close_Breaker/1 -> Three-Phase Breaker/1
  Vabcref/1 -> Demux2/1
  Demux2/1 -> Controlled Voltage Source/1  "Va"
  Demux2/2 -> Controlled Voltage Source1/1  "Vb"
  Demux2/3 -> Controlled Voltage Source2/1  "Vc"
  Constant/1 -> LSC/2
  Constant1/1 -> Switch/3
  Constant2/1 -> Switch/1
  Switch/1 -> Three-Phase Breaker1/1
  Constant4/1 -> Switch1/1
  Constant3/1 -> Switch1/3
  Switch1/1 -> Three-Phase Breaker2/1
  0=Avg_1=Switch/1 -> Switch1/2, Switch/2
  connections:
  La_DVR1/LConn1 -- INV/RConn1
  LV/RConn1 -- Three-Phase Transformer (Two Windings)/RConn1 -- High Res Grounding/LConn1
  La_DVR1/RConn1 -- La_DVR4/RConn1 -- LV/LConn1
  LSC/LConn3 -- Three-Phase Breaker1/RConn3
  Three-Phase Transformer (Two Windings)/LConn3 -- HV/LConn3
  LSC/LConn2 -- Three-Phase Breaker1/RConn2
  Three-Phase Transformer (Two Windings)/RConn3 -- LV/RConn3 -- High Res Grounding/LConn3
  La_DVR2/RConn1 -- La_DVR5/RConn1 -- LV/LConn2
  Three-Phase Transformer (Two Windings)/LConn2 -- HV/LConn2
  LSC/RConn2 -- INV_DClink/RConn2
  LSC/LConn1 -- Three-Phase Breaker1/RConn1
  LSC/RConn1 -- INV_DClink/RConn1
  Three-Phase Transformer (Two Windings)/RConn2 -- LV/RConn2 -- High Res Grounding/LConn2
  "\tP"/RConn1 -- INV_DClink/LConn1
  Three-Phase Transformer (Two Windings)/LConn1 -- HV/LConn1
  LV/LConn3 -- La_DVR3/RConn1 -- La_DVR6/RConn1
  La_DVR3/LConn1 -- INV/RConn3
  La_DVR5/LConn1 -- La_DVR6/LConn1 -- La_DVR4/LConn1
  La_DVR2/LConn1 -- INV/RConn2
  INV_DClink/LConn2 -- M/RConn1
  Three-Phase Breaker/LConn2 -- B/RConn1
  Three-Phase Breaker/RConn2 -- HV/RConn2
  HV/RConn3 -- Three-Phase Breaker/RConn3
  Three-Phase Breaker/LConn3 -- C/RConn1
  HV/RConn1 -- Three-Phase Breaker/RConn1
  Three-Phase Breaker/LConn1 -- A/RConn1
  Controlled Voltage Source2/LConn1 -- Controlled Voltage Source/LConn1 -- Controlled Voltage Source1/LConn1
  Three-Phase Breaker1/LConn1 -- Three-Phase Breaker2/LConn1 -- INV/LConn1
  Three-Phase Breaker1/LConn2 -- Three-Phase Breaker2/LConn2 -- INV/LConn2
  Three-Phase Breaker1/LConn3 -- Three-Phase Breaker2/LConn3 -- INV/LConn3
  Three-Phase Breaker2/RConn1 -- Controlled Voltage Source/RConn1
  Controlled Voltage Source1/RConn1 -- Three-Phase Breaker2/RConn2
  Controlled Voltage Source2/RConn1 -- Three-Phase Breaker2/RConn3

== system pwrsys/Voltage Sources/SM_TG_EXC ==
  note: Measurements
  note: Datalog
  Psp : Inport
  Vsp : Inport  Port=2
  PSS : Inport  Port=3
  Bus Creator : BusCreator  Inputs=10
  Bus Selector : BusSelector  OutputSignals="Mechanical.Rotor speed  wm  (pu),dq0 components.Stator voltage  vq (pu),dq0 components.Stator voltage  vd (pu),Output active power   Peo (pu),Output reactive power  Qeo (pu),dq0 components.Field current  ifd (pu),Load angle   delta  (deg),Mechanical.Rotor speed deviation  dw (pu),Mechanical.Rotor mechanical angle  theta (deg)"
  Controllers : Subsystem  SystemSampleTime=1/(20*grid.fn)
  GT SM : powerlib/Machines/Synchronous Machine pu Standard  PresetModel=No  MechanicalLoad=Mechanical power Pm  ShowDetailedParameters=on  RotorType=Salient-pole  Units=per unit standard parameters  MeasurementBus=off  NominalParameters=[SMPn SMVn SMfn]  Reactances1=[ 2.12, 0.299, 0.188, 1.76, 0.65, 0.25, 0.15 ]  Reactances2=[SMXd SMXdp SMXdpp SMXq SMXqpp SMXl]  dAxisTimeConstants=Short-circuit  qAxisTimeConstants=Short-circuit  TimeConstants1="[ 4.4849  0.0681  0.1  ]"  TimeConstants2=[ 8.0, 0.03, 1.0, 0.07 ]  TimeConstants3="[  4.49  0.0681  0.0513  ]"  TimeConstants4=[ 8.0, 0.03, 0.3371, 0.0295 ]  TimeConstants5=[ 1.01, 0.053, 0.1 ]  TimeConstants6=[ 1.3201, 0.023, 1.0, 0.07 ]  TimeConstants7=[SMTdpSC SMTdppSC SMTqppSC]  TimeConstants8=[ 1.3201, 0.0231, 0.3371, 0.0295 ]  StatorResistance=SMRs  Mechanical=[SMM 0 SMp]  PolePairs=20  InitialConditions=[0 -65.6047 0.526967 0.526967 0.526967 -11.262 -131.262 108.738 (3/2)^0.5*1.57232]  SetSaturation=on  Saturation=[0.6404,0.7127,0.8441,0.9214,0.9956,1.082,1.19,1.316,1.457;0.7,0.7698,0.8872,0.9466,0.9969,1.046,1.1,1.151,1.201]  LoadFlowParameters=[2 44600000 0 0 0]  TsPowergui=0  TsBlock=-1  IterativeModel=Trapezoidal non iterative  IterativeDiscreteModel=Trapezoidal non iterative  BusType=swing  Pref=0  Qref=0  Qmin=-inf  Qmax=inf  PLF=0  QLF=0
      settings: SourceProductName=Simscape Power Systems
  GT_BUS : powerlib/Measurements/Three-Phase V-I Measurement  VoltageMeasurement=phase-to-ground  SetLabelV=off  LabelV=vconv  Vpu=off  VpuLL=off  CurrentMeasurement=yes  SetLabelI=off  LabelI=iconv  Ipu=off  Pbase=sn  Vbase=uab  OutputType=Complex  PhasorSimulation=off  PSBequivalent=0
  Hypot : Math  Operator=hypot  SaturateOnIntegerOverflow=on
  Low-pass filter : DiscreteIntegrator  gainval=3/ExcTr  InitialCondition=1  SampleTime=SIMU.Ts  UpperSaturationLimit=Refmax/Kp  LowerSaturationLimit=Refmin/Kp  ICPrevOutput=DiscIntNeverNeededParam  ICPrevScaledInput=DiscIntNeverNeededParam
  Sum3 : Sum  Inputs=-+
  Sum6 : Sum  Inputs=-+
  w ref pu : Constant
  A : PMIOPort  Side=Right
  B : PMIOPort  Port=2  Side=Right
  C : PMIOPort  Port=3  Side=Right
  m : Outport
  wires:
  [we] -> Sum6/2
  w ref pu/1 -> Sum6/1
  Bus Selector/6 -> [Ifd]  "<Field current  ifd (pu)>"
  GT SM/1 -> Bus Selector/1
  Bus Selector/5 -> [Qac]  "<Output reactive power  Qeo (pu)>"
  Bus Selector/3 -> Hypot/2  "<Stator voltage  vd (pu)>"
  Bus Selector/2 -> Hypot/1  "<Stator voltage  vq (pu)>"
  Bus Selector/1 -> [we]  "<Rotor speed  wm  (pu)>"
  Bus Selector/4 -> [Pac]  "<Output active power   Peo (pu)>"
  [Vavg] -> Bus Creator/4  "Vavg"
  [Pac] -> Bus Creator/1  "Pel"
  [Qac] -> Bus Creator/2  "Q"
  [we] -> Bus Creator/3  "w"
  [Ifd] -> Bus Creator/5  "Ifd"
  [Vfd] -> Bus Creator/6  "Vfd"
  Bus Creator/1 -> m/1  "GT"
  Sum6/1 -> Controllers/1(deltaw)  "dwe"
  Psp/1 -> Controllers/2(Psp)  "Psp"
  Vsp/1 -> Controllers/3(Vref)
  [Vavg] -> Controllers/4(Vm)  "Vavg"
  [Ifd] -> Controllers/5(Ifd)  "Ifd"
  [Pm] -> Bus Creator/7  "Pm"
  Controllers/2(Efd) -> [Vfd], GT SM/2
  Controllers/1(Pm) -> [Pm], GT SM/1
  Low-pass filter/1 -> [Vavg], Sum3/1  "Vavg_pu"
  Sum3/1 -> Low-pass filter/1
  Hypot/1 -> Sum3/2
  GT_BUS/1 -> [Vabc]
  GT_BUS/2 -> [Iabc]
  Bus Selector/7 -> [delta]  "<Load angle   delta  (deg)>"
  Bus Selector/8 -> [dw]  "<Rotor speed deviation  dw (pu)>"
  Bus Selector/9 -> [theta]  "<Rotor mechanical angle  theta (deg)>"
  [theta] -> Bus Creator/10  "theta"
  [dw] -> Bus Creator/9  "dw"
  [delta] -> Bus Creator/8  "delta"
  PSS/1 -> Controllers/6(PSS)
  connections:
  B/RConn1 -- GT_BUS/RConn2
  A/RConn1 -- GT_BUS/RConn1
  C/RConn1 -- GT_BUS/RConn3
  GT_BUS/LConn1 -- GT SM/RConn1
  GT_BUS/LConn2 -- GT SM/RConn2
  GT_BUS/LConn3 -- GT SM/RConn3
